simulink model "locationStorage"  (R2023a)
settings: Solver=VariableStepAuto  StartTime=0.0  StopTime=10.0  RelTol=1e-3
values from neighbouring files (symbols this model uses):
  axleLength = 0.136    [robotParameters.m]
  distanceSimulated = 1    [robotParameters.m]
  ticksPerRot = 20    [robotParameters.m]
  wheelR = 0.031    [robotParameters.m]
libraries: mobileRoboticsTrainingLib x1
settings Model: Creator=friso  LastModifiedBy=friso

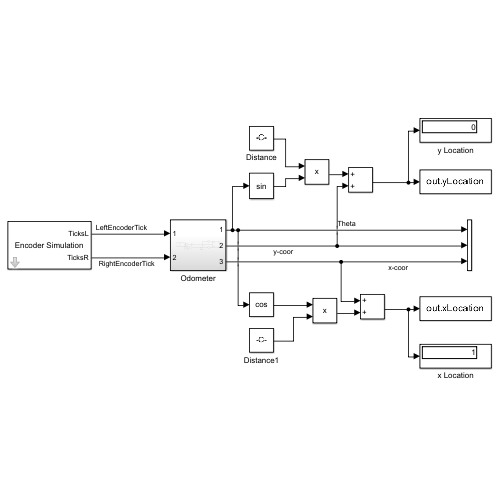
[thumbnail: Simulink's stored preview of the top-level diagram]
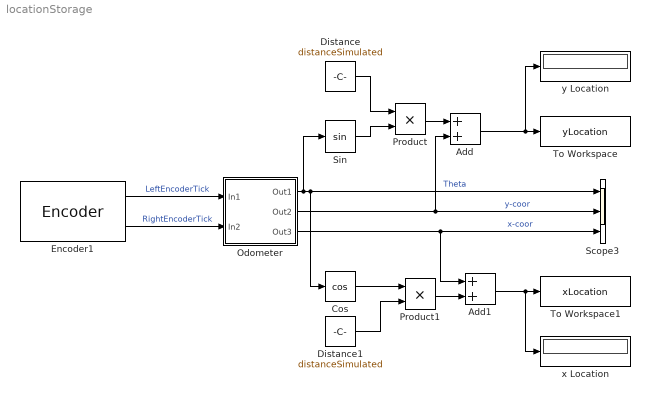
== system locationStorage ==
  Add : Sum
  Add1 : Sum
  Cos : Trigonometry  Operator=cos
  Distance : Constant  Value=distanceSimulated
  Distance1 : Constant  Value=distanceSimulated
  Encoder1 : mobileRoboticsTrainingLib/Encoder  axleLength=axleLength  wheelR=wheelR  ticksPerRot=ticksPerRot
      settings: SourceProductName=Mobile Robotics Training Library
  Odometer : Subsystem
  Product : Product
  Product1 : Product
  Scope3 : Scope  NumInputPorts=3
  Sin : Trigonometry
  To Workspace : ToWorkspace  VariableName=yLocation  SaveFormat=Timeseries  SampleTime=-1
  To Workspace1 : ToWorkspace  VariableName=xLocation  SaveFormat=Timeseries  SampleTime=-1
  x Location : Display
  y Location : Display
  wires:
  Encoder1/2 -> Odometer/2(In2)  "RightEncoderTick"
  Odometer/1(Out1) -> Cos/1, Scope3/1, Sin/1  "Theta"
  Odometer/2(Out2) -> Add/2, Scope3/2  "y-coor"
  Encoder1/1 -> Odometer/1(In1)  "LeftEncoderTick"
  Odometer/3(Out3) -> Add1/1, Scope3/3  "x-coor"
  Distance/1 -> Product/1
  Sin/1 -> Product/2
  Cos/1 -> Product1/1
  Distance1/1 -> Product1/2
  Product/1 -> Add/1
  Product1/1 -> Add1/2
  Add/1 -> y Location/1, To Workspace/1
  Add1/1 -> x Location/1, To Workspace1/1

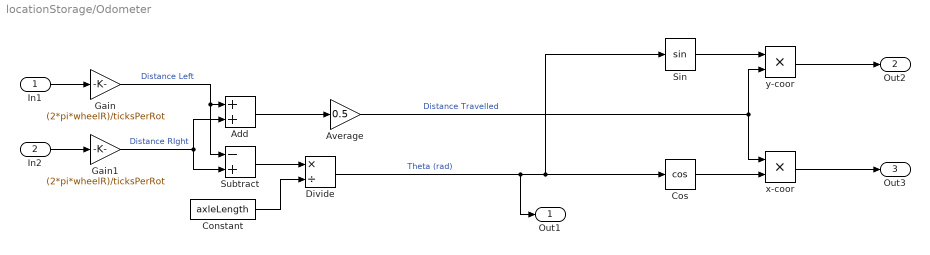
== system locationStorage/Odometer ==
  In1 : Inport
  In2 : Inport  Port=2
  Add : Sum
  Average : Gain  Gain=0.5
  Constant : Constant  Value=axleLength
  Cos : Trigonometry  Operator=cos  OutputSignalType=real
  Divide : Product  Inputs=*/
  Gain : Gain  Gain=(2*pi*wheelR)/ticksPerRot
  Gain1 : Gain  Gain=(2*pi*wheelR)/ticksPerRot
  Sin : Trigonometry  OutputSignalType=real
  Subtract : Sum  Inputs=-+
  x-coor : Product
  y-coor : Product
  Out1 : Outport
  Out2 : Outport  Port=2
  Out3 : Outport  Port=3
  wires:
  x-coor/1 -> Out3/1
  Divide/1 -> Out1/1, Sin/1, Cos/1  "Theta (rad)"
  Gain/1 -> Subtract/1, Add/1  "Distance Left"
  In1/1 -> Gain/1
  Cos/1 -> x-coor/2
  Subtract/1 -> Divide/1
  Add/1 -> Average/1
  Average/1 -> x-coor/1, y-coor/2  "Distance Travelled"
  Gain1/1 -> Add/2, Subtract/2  "Distance RIght"
  Sin/1 -> y-coor/1
  In2/1 -> Gain1/1
  Constant/1 -> Divide/2
  y-coor/1 -> Out2/1
